simulink model "Control_project_variable_gain"  (R2016a)
settings: Solver=VariableStepAuto  StartTime=0.0  StopTime=10  RelTol=1e-3
libraries: simulink x6
settings Model: Creator=User  LastModifiedBy=User

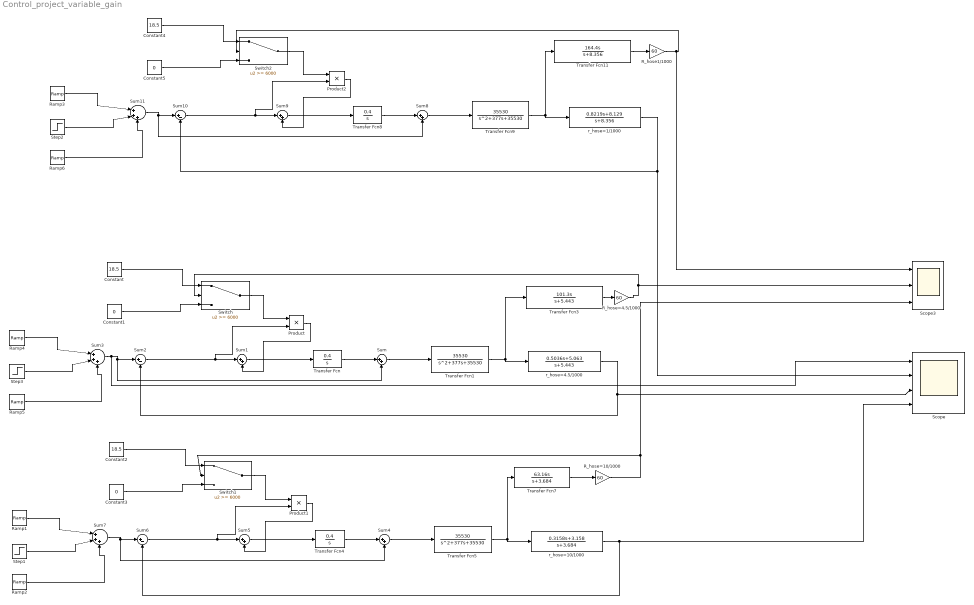
== system Control_project_variable_gain ==
  Constant : Constant  Value=18.5
  Constant1 : Constant  Value=0
  Constant2 : Constant  Value=18.5
  Constant3 : Constant  Value=0
  Constant4 : Constant  Value=18.5
  Constant5 : Constant  Value=0
  Product : Product
  Product1 : Product
  Product2 : Product
  R_hose1/1000 : Gain  Gain=60
  R_hose=10/1000 : Gain  Gain=60
  R_hose=4.5/1000 : Gain  Gain=60
  Ramp1 : simulink/Sources/Ramp  slope=100  start=1  X0=0
  Ramp2 : simulink/Sources/Ramp  slope=-100  start=1.15  X0=0
  Ramp3 : simulink/Sources/Ramp  slope=100  start=1  X0=0
  Ramp4 : simulink/Sources/Ramp  slope=100  start=1  X0=0
  Ramp5 : simulink/Sources/Ramp  slope=-100  start=1.15  X0=0
  Ramp6 : simulink/Sources/Ramp  slope=-100  start=1.15  X0=0
  Scope : Scope  NumInputPorts=4
  Scope3 : Scope  NumInputPorts=3
  Step1 : Step  Time=5  After=-15  SampleTime=0
  Step2 : Step  Time=5  After=-15  SampleTime=0
  Step3 : Step  Time=5  After=-15  SampleTime=0
  Sum{,1,4..5,8..9} (6 alike) : Sum  Inputs=|++
  Sum10 : Sum  Inputs=|+-
  Sum11 : Sum  Inputs=|+++
  Sum2 : Sum  Inputs=|+-
  Sum3 : Sum  Inputs=|+++
  Sum6 : Sum  Inputs=|+-
  Sum7 : Sum  Inputs=|+++
  Switch : Switch  Threshold=6000
  Switch1 : Switch  Threshold=6000
  Switch2 : Switch  Threshold=6000
  Transfer Fcn : TransferFcn  Numerator=[0.4]  Denominator=[1 0]
  Transfer Fcn1 : TransferFcn  Numerator=[35530]  Denominator="[1  377 35530]"
  Transfer Fcn11 : TransferFcn  Numerator=[164.4 0]  Denominator=[1 8.356]
  Transfer Fcn3 : TransferFcn  Numerator=[101.3 0]  Denominator=[1 5.443]
  Transfer Fcn4 : TransferFcn  Numerator=[0.4]  Denominator=[1 0]
  Transfer Fcn5 : TransferFcn  Numerator=[35530]  Denominator="[1  377 35530]"
  Transfer Fcn7 : TransferFcn  Numerator=[63.16 0]  Denominator=[1 3.684]
  Transfer Fcn8 : TransferFcn  Numerator=[0.4]  Denominator=[1 0]
  Transfer Fcn9 : TransferFcn  Numerator=[35530]  Denominator="[1  377 35530]"
  r_hose=1/1000 : TransferFcn  Numerator=[0.8219 8.129]  Denominator=[1 8.356]
  r_hose=10/1000 : TransferFcn  Numerator=[0.3158 3.158]  Denominator=[1 3.684]
  r_hose=4.5/1000 : TransferFcn  Numerator=[0.5036 5.063]  Denominator=[1 5.443]
  wires:
  Transfer Fcn/1 -> Sum/1
  Transfer Fcn1/1 -> r_hose=4.5/1000/1, Transfer Fcn3/1
  Sum/1 -> Transfer Fcn1/1
  Sum2/1 -> Product/2, Sum1/1
  Constant/1 -> Switch/1
  Constant1/1 -> Switch/3
  Sum1/1 -> Transfer Fcn/1
  Switch/1 -> Product/1
  Product/1 -> Sum1/2
  r_hose=4.5/1000/1 -> Sum2/2, Scope/3
  Transfer Fcn3/1 -> R_hose=4.5/1000/1
  Step3/1 -> Sum3/2
  Ramp4/1 -> Sum3/1
  Ramp5/1 -> Sum3/3
  Sum3/1 -> Scope/1, Sum/2, Sum2/1
  Transfer Fcn4/1 -> Sum4/1
  Transfer Fcn5/1 -> r_hose=10/1000/1, Transfer Fcn7/1
  Sum4/1 -> Transfer Fcn5/1
  Sum6/1 -> Product1/2, Sum5/1
  Constant2/1 -> Switch1/1
  Constant3/1 -> Switch1/3
  Sum5/1 -> Transfer Fcn4/1
  Switch1/1 -> Product1/1
  Product1/1 -> Sum5/2
  r_hose=10/1000/1 -> Sum6/2, Scope/4
  Transfer Fcn7/1 -> R_hose=10/1000/1
  Step1/1 -> Sum7/2
  Ramp1/1 -> Sum7/1
  Ramp2/1 -> Sum7/3
  Sum7/1 -> Sum4/2, Sum6/1
  Transfer Fcn8/1 -> Sum8/1
  Transfer Fcn9/1 -> r_hose=1/1000/1, Transfer Fcn11/1
  Sum8/1 -> Transfer Fcn9/1
  Sum10/1 -> Product2/2, Sum9/1
  Constant4/1 -> Switch2/1
  Constant5/1 -> Switch2/3
  Sum9/1 -> Transfer Fcn8/1
  Switch2/1 -> Product2/1
  Product2/1 -> Sum9/2
  r_hose=1/1000/1 -> Scope/2, Sum10/2
  Transfer Fcn11/1 -> R_hose1/1000/1
  Step2/1 -> Sum11/2
  Ramp3/1 -> Sum11/1
  Ramp6/1 -> Sum11/3
  Sum11/1 -> Sum8/2, Sum10/1
  R_hose1/1000/1 -> Scope3/1, Switch2/2
  R_hose=4.5/1000/1 -> Scope3/2, Switch/2
  R_hose=10/1000/1 -> Scope3/3, Switch1/2
